simulink model "linear_model_saturday"  (R2025a)
settings: Solver=VariableStepAuto  StartTime=0.0  StopTime=10  RelTol=1e-3
model workspace: external: MATLAB File C:\Users\josep\Documents\mecatro_mines_05\matlab\linear_model_constants.m (data not in the file)
values from neighbouring files (symbols this model uses):
  A = inv(T) * Q_0    [linear_model_constants.m]
  A_W = [0 1 0 ... (first row only)    [linear_model_constants.m]
  B = inv(T) * Q_1    [linear_model_constants.m]
  B_W = [-d_i 0 ... (first row only)    [linear_model_constants.m]
  C_W = [2/rho 0 -2]    [linear_model_constants.m]
  d_i = 0.100    (= 0.1)    [linear_model_constants.m]
  g = 9.81    [linear_model_constants.m]
  L = place(A_W', C_W', p_L)'    [linear_model_constants.m]
settings Model: Creator=josep  LastModifiedBy=josep

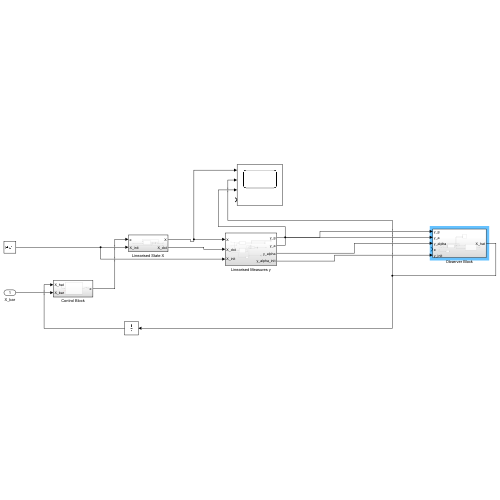
[thumbnail: Simulink's stored preview of the top-level diagram]
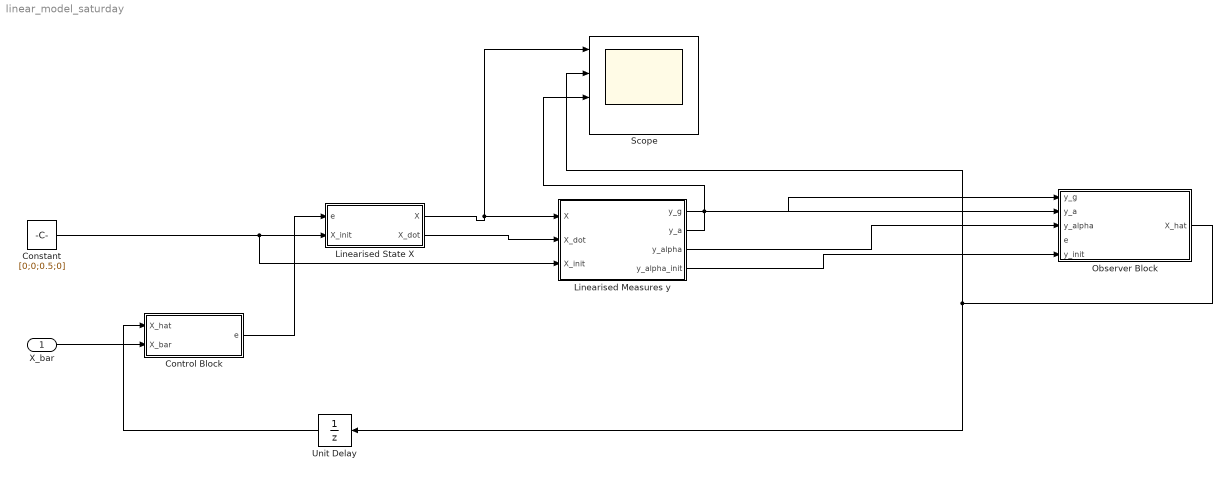
== system linear_model_saturday ==
  X_bar : Inport
  Constant : Constant  Value=[0;0;0.5;0]
  Control Block : Subsystem
  Linearised Measures y : Subsystem
  Linearised State X : Subsystem
  Observer Block : Subsystem
  Scope : Scope  NumInputPorts=4
      settings: ActiveDisplayYMinimum=-35.741935898306792  ActiveDisplayYMaximum=11.265008746360857
  Unit Delay : UnitDelay  SampleTime=0.01  HasFrameUpgradeWarning=on
  wires:
  Linearised State X/1(X) -> Scope/1, Linearised Measures y/1(X)
  Linearised Measures y/1(y_g) -> Observer Block/1(y_g)
  Linearised Measures y/3(y_alpha) -> Observer Block/3(y_alpha)
  Linearised Measures y/2(y_a) -> Scope/3, Observer Block/2(y_a)
  X_bar/1 -> Control Block/2(X_bar)
  Unit Delay/1 -> Control Block/1(X_hat)
  Linearised State X/2(X_dot) -> Linearised Measures y/2(X_dot)
  Constant/1 -> Linearised Measures y/3(X_init), Linearised State X/2(X_init)
  Observer Block/1(X_hat) -> Scope/2, Unit Delay/1
  Control Block/1(e) -> Linearised State X/1(e)
  Linearised Measures y/4(y_alpha_init) -> Observer Block/5(y_init)

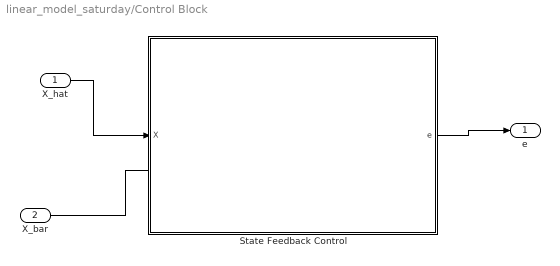
== system linear_model_saturday/Control Block ==
  X_hat : Inport
  X_bar : Inport  Port=2
  State Feedback Control : MATLAB Function  TreatAsAtomicUnit=on
  e : Outport
  wires:
  X_hat/1 -> State Feedback Control/1(X)
  X_bar/1 -> ?
  State Feedback Control/1(e) -> e/1

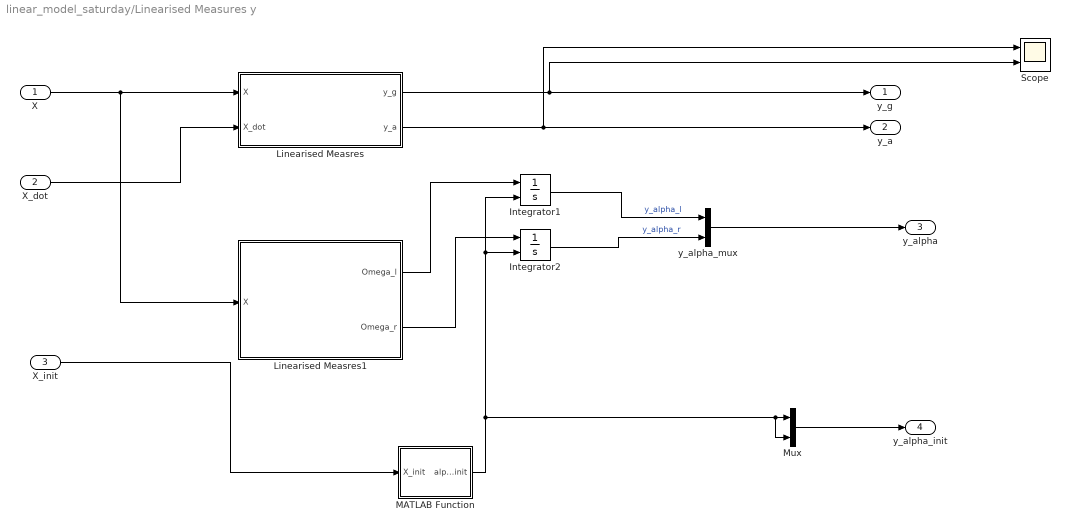
== system linear_model_saturday/Linearised Measures y ==
  X : Inport
  X_dot : Inport  Port=2
  X_init : Inport  Port=3
  Integrator1 : Integrator  InitialConditionSource=external
  Integrator2 : Integrator  InitialConditionSource=external
  Linearised Measres : MATLAB Function  TreatAsAtomicUnit=on
  Linearised Measres1 : MATLAB Function  TreatAsAtomicUnit=on
  MATLAB Function : MATLAB Function  TreatAsAtomicUnit=on
  Mux : Mux  Inputs=2
  Scope : Scope  NumInputPorts=2
      settings: ActiveDisplayYMinimum=-0.51043745646463368  ActiveDisplayYMaximum=1.2338081847305338  DataLoggingVariableName=ScopeData2
  y_alpha_mux : Mux  Inputs=2
  y_g : Outport  PortDimensions=3
  y_a : Outport  Port=2
  y_alpha : Outport  Port=3
  y_alpha_init : Outport  Port=4
  wires:
  X/1 -> Linearised Measres1/1(X), Linearised Measres/1(X)
  Linearised Measres/2(y_a) -> y_a/1, Scope/1
  Linearised Measres/1(y_g) -> y_g/1, Scope/2
  y_alpha_mux/1 -> y_alpha/1
  Linearised Measres1/1(Omega_l) -> Integrator1/1
  Integrator1/1 -> y_alpha_mux/1  "y_alpha_l"
  Linearised Measres1/2(Omega_r) -> Integrator2/1
  Integrator2/1 -> y_alpha_mux/2  "y_alpha_r"
  X_dot/1 -> Linearised Measres/2(X_dot)
  X_init/1 -> MATLAB Function/1(X_init)
  MATLAB Function/1(alpha_init) -> Mux/2, Mux/1, Integrator2/2, Integrator1/2
  Mux/1 -> y_alpha_init/1

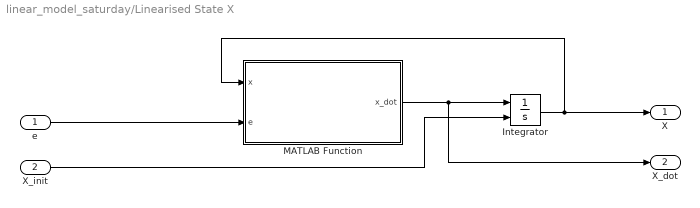
== system linear_model_saturday/Linearised State X ==
  e : Inport  PortDimensions=2
  X_init : Inport  Port=2  PortDimensions=4
  Integrator : Integrator  InitialConditionSource=external
  MATLAB Function : MATLAB Function  TreatAsAtomicUnit=on
  X : Outport  PortDimensions=4
  X_dot : Outport  Port=2  PortDimensions=4
  wires:
  e/1 -> MATLAB Function/2(e)
  MATLAB Function/1(x_dot) -> X_dot/1, Integrator/1
  Integrator/1 -> MATLAB Function/1(x), X/1
  X_init/1 -> Integrator/2

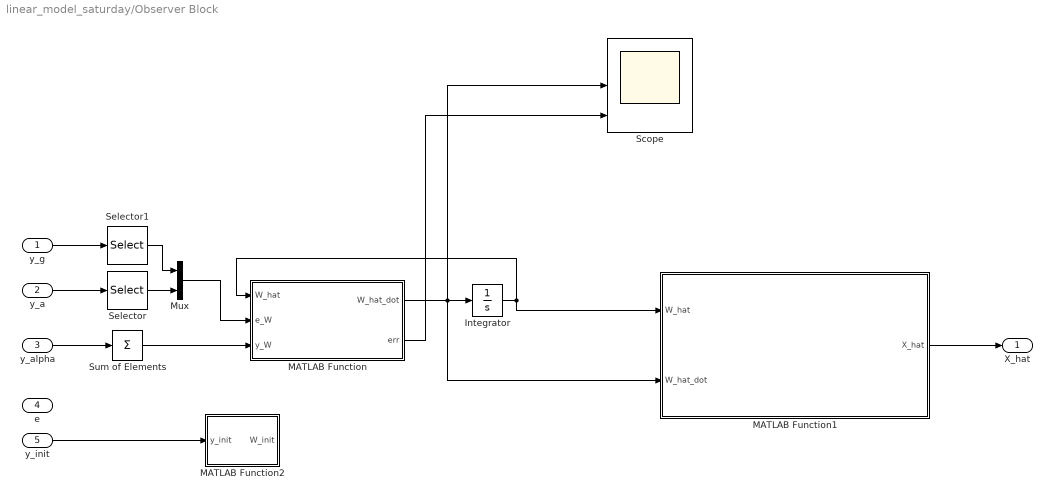
== system linear_model_saturday/Observer Block ==
  y_g : Inport  PortDimensions=3
  y_a : Inport  Port=2
  y_alpha : Inport  Port=3  PortDimensions=2
  e : Inport  Port=4
  y_init : Inport  Port=5  PortDimensions=4
  Integrator : Integrator  InitialCondition=[0; 0; 0]
  MATLAB Function : MATLAB Function  TreatAsAtomicUnit=on
  MATLAB Function1 : MATLAB Function  TreatAsAtomicUnit=on
  MATLAB Function2 : MATLAB Function  TreatAsAtomicUnit=on
  Mux : Mux  Inputs=2
  Scope : Scope  NumInputPorts=3
      settings: ActiveDisplayYMinimum=-9.354319725259022E-9  ActiveDisplayYMaximum=1.5615645358879332E-8
  Selector : Selector  InputPortWidth=3  IndexOptions=Index vector (dialog)  Indices=1  OutputSizes=1
  Selector1 : Selector  InputPortWidth=3  IndexOptions=Index vector (dialog)  Indices=2  OutputSizes=1
  Sum of Elements : Sum  Inputs=+
  X_hat : Outport  PortDimensions=4
  wires:
  MATLAB Function/1(W_hat_dot) -> MATLAB Function1/2(W_hat_dot), Integrator/1, Scope/2
  Integrator/1 -> MATLAB Function1/1(W_hat), MATLAB Function/1(W_hat)
  MATLAB Function1/1(X_hat) -> X_hat/1
  y_a/1 -> Selector/1
  y_g/1 -> Selector1/1
  y_alpha/1 -> Sum of Elements/1
  Selector1/1 -> Mux/1
  Selector/1 -> Mux/2
  Mux/1 -> MATLAB Function/2(e_W)
  y_init/1 -> MATLAB Function2/1(y_init)
  Sum of Elements/1 -> MATLAB Function/3(y_W)
  MATLAB Function/2(err) -> Scope/3

== matlab function linear_model_saturday/Linearised Measures y/Linearised Measres ==
  data: X input; y_g output; y_a output; X_dot input; g parameter; d_i parameter
function [y_g, y_a] = lin_y(X, X_dot, g, d_i)

% y_g is the 3 dimensional output that is given by C_1 X + b_1
% y_a is the 3 dimensional output, that is given by C_2 X + b_2

y_g = [0
       X(4)
       0];


y_a = [X_dot(2) - g * X(3) + d_i * X_dot(4)
       0
       0];

== matlab function linear_model_saturday/Linearised State X/MATLAB Function ==
  data: x input; x_dot output; e input; A parameter; B parameter
function x_dot = lin_state_eqn(x, e, A, B)
    % e is the 2d control input dU_l and dU_r,
    % where in the cascade equation it is used as (dU_l + dU_r)
    x_dot = A * x + B * e;
end

== matlab function linear_model_saturday/Linearised Measures y/Linearised Measres1 ==
  data: X input; Omega_l output; Omega_r output; rho parameter
function [Omega_l, Omega_r] = lin_Omega(X, rho)

Omega_lr = X(2)/rho - X(4);
Omega_l = Omega_lr;
Omega_r = Omega_lr;

== matlab function linear_model_saturday/Observer Block/MATLAB Function ==
  data: W_hat input; e_W input; y_W input; W_hat_dot output size=3; A_W parameter; C_W parameter; B_W parameter; L parameter; err output
function [W_hat_dot, err] = observer(W_hat, e_W, y_W, A_W, C_W, B_W, L)

% Write the observer equation out, W_hat_dot = A * W_hat + B * e + L (y -
% y_hat) where e is a 2d vector as a linear combination of y_g and y_a




y_hat = C_W * W_hat;

err = y_W - y_hat;
W_hat_dot = A_W * W_hat + B_W * e_W + (y_W - y_hat) * L;

== matlab function linear_model_saturday/Observer Block/MATLAB Function1 ==
  data: W_hat input; X_hat output; W_hat_dot input
function X_hat = W_hat_to_X_hat(W_hat, W_hat_dot)

X_hat = [W_hat(1)
         W_hat_dot(1)
         W_hat(3)
         W_hat_dot(3)];

== matlab function linear_model_saturday/Control Block/State Feedback Control ==
  data: X input; e output; K parameter
function e = state_feedback(X, K)
    % Function that gives the control signal for the eqn
    % X_dot = (A - BK)X + Bkr, where u = -KX + r, where r is
    % a reference consant (or non constant maybe ?)
    
    % solving the system, we get that equilibrium will be reached at x_bar =
    % - (A - BK)^-1 Br, which means that if we set a reference r, we can control
    % where the system stabilises to. Thus, r = (K - B^-1 A)x_bar
    
    % the control signal "u" here is given by the sum of components of e, so e
    % should be 
    
      e_unlimited = - K * X;
      e = [min(max(e_unlimited(1), -12), 12)
           min(max(e_unlimited(2), -12), 12)];
end

== matlab function linear_model_saturday/Observer Block/MATLAB Function2 ==
  data: y_init input; W_init output; d_i parameter
function W_init = W_init(y_init, d_i)

W_init = [y_init(1) + y_init(2)
          0
          0];

== matlab function linear_model_saturday/Linearised Measures y/MATLAB Function ==
  data: X_init input; alpha_init output; rho parameter
function alpha_init = alpha_init(X_init, rho)

alpha_init = X_init(1) / rho - X_init(3);
